simulink model "newdesign"  (R2017b)
settings: Solver=VariableStepAuto  StartTime=0.0  StopTime=inf  RelTol=1e-3
settings Model: Creator=E6320  LastModifiedBy=E6320

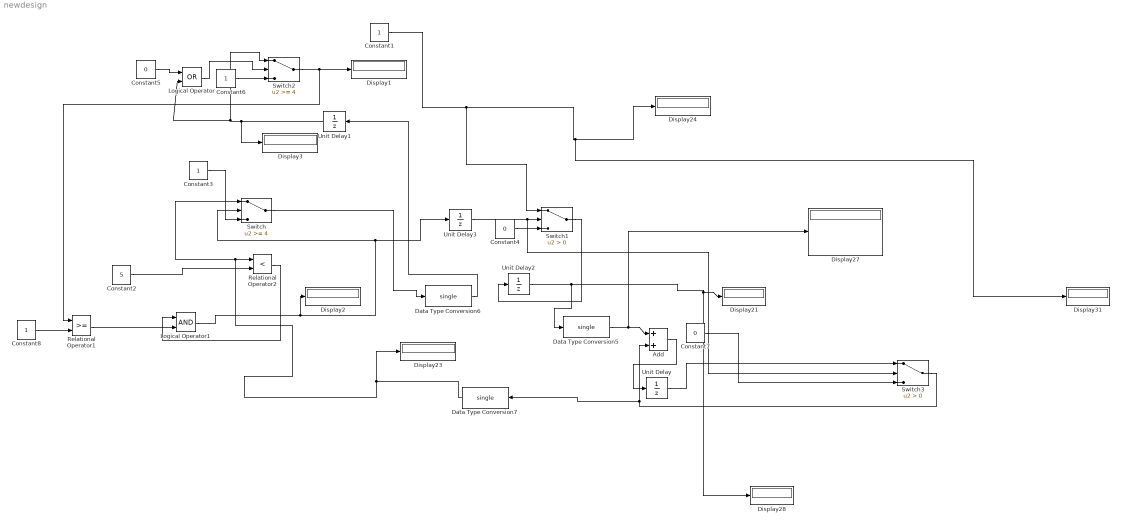
== system newdesign ==
  Add : Sum  OutDataTypeStr=single
  Constant{1,3,6,8} (4 alike) : Constant  OutDataTypeStr=single
  Constant2 : Constant  Value=5  OutDataTypeStr=single
  Constant4 : Constant  Value=0  OutDataTypeStr=single
  Constant5 : Constant  Value=0  OutDataTypeStr=single
  Constant7 : Constant  Value=0  OutDataTypeStr=single
  Data Type Conversion5 : DataTypeConversion  OutDataTypeStr=single
  Data Type Conversion6 : DataTypeConversion  OutDataTypeStr=single  RndMeth=Round
  Data Type Conversion7 : DataTypeConversion  OutDataTypeStr=single  RndMeth=Ceiling
  Display{1..3,21,23..24,27..28,31} (9 alike) : Display
  Logical Operator : Logic  Operator=OR  AllPortsSameDT=off  OutDataTypeStr=boolean
  Logical Operator1 : Logic  AllPortsSameDT=off  OutDataTypeStr=boolean
  Relational Operator1 : RelationalOperator  OutDataTypeStr=boolean  ZeroCross=off  RndMeth=Simplest
  Relational Operator2 : RelationalOperator  Operator=<  OutDataTypeStr=boolean  ZeroCross=off  RndMeth=Simplest
  Switch : Switch  Threshold=4
  Switch1 : Switch  Criteria=u2 > Threshold
  Switch2 : Switch  Threshold=4
  Switch3 : Switch  Criteria=u2 > Threshold
  Unit Delay : UnitDelay  InputProcessing=Columns as channels (frame based)  SampleTime=10
  Unit Delay1 : UnitDelay  InputProcessing=Columns as channels (frame based)  SampleTime=0.1
  Unit Delay2 : UnitDelay  InputProcessing=Columns as channels (frame based)  SampleTime=0.1
  Unit Delay3 : UnitDelay  InputProcessing=Columns as channels (frame based)  SampleTime=0.1
  wires:
  Unit Delay2/1 -> Data Type Conversion5/1, Display21/1, Display28/1
  Data Type Conversion6/1 -> Unit Delay1/1
  Data Type Conversion5/1 -> Display27/1, Add/1
  Constant2/1 -> Relational Operator2/2
  Constant3/1 -> Switch/3
  Switch/1 -> Data Type Conversion6/1
  Switch1/1 -> Unit Delay2/1
  Constant4/1 -> Switch1/3
  Constant1/1 -> Switch1/1, Display31/1, Display24/1
  Constant5/1 -> Logical Operator/1
  Logical Operator/1 -> Switch2/2
  Constant6/1 -> Switch2/3
  Unit Delay1/1 -> Display3/1, Switch2/1, Logical Operator/2
  Unit Delay3/1 -> Switch3/2, Switch1/2
  Data Type Conversion7/1 -> Relational Operator2/1, Switch/1, Display23/1
  Constant7/1 -> Switch3/3
  Unit Delay/1 -> Switch3/1
  Logical Operator1/1 -> Display2/1, Unit Delay3/1, Switch/2
  Relational Operator2/1 -> Logical Operator1/1
  Switch2/1 -> Relational Operator1/1, Display1/1
  Relational Operator1/1 -> Logical Operator1/2
  Constant8/1 -> Relational Operator1/2
  Add/1 -> Unit Delay/1
  Switch3/1 -> Data Type Conversion7/1, Add/2
